simulink model "gm_flightController"  (R2018b)
settings: Solver=ode3  StartTime=0  StopTime=TFinal  FixedStep=Ts  RelTol=1e-3  EnableMultiTasking=on
libraries: hdlmdlgenlib x14
(part 2 of 2)

== system gm_flightController/Flight Controller/Yaw/Sum2 ==
  In1 : Inport
  In2 : Inport  Port=2
  Sum2 : Sum  Inputs=+-  OutDataTypeStr=single  SampleTime=0.005  SaturateOnIntegerOverflow=on  InputSameDT=on
  Out1 : Outport
  wires:
  In1/1 -> Sum2/1
  In2/1 -> Sum2/2
  Sum2/1 -> Out1/1

== system gm_flightController/Flight Controller/gravity feedforward//equilibrium thrust/D_z ==
  In1 : Inport
  In2 : Inport  Port=2
  D_z : Product  Inputs=**  OutDataTypeStr=single  SampleTime=0.005  SaturateOnIntegerOverflow=on
  Out1 : Outport
  wires:
  In1/1 -> D_z/1
  In2/1 -> D_z/2
  D_z/1 -> Out1/1

== system gm_flightController/Flight Controller/gravity feedforward//equilibrium thrust/P_z ==
  In1 : Inport
  In2 : Inport  Port=2
  P_z : Product  Inputs=**  OutDataTypeStr=single  SampleTime=0.005  SaturateOnIntegerOverflow=on
  Out1 : Outport
  wires:
  In1/1 -> P_z/1
  In2/1 -> P_z/2
  P_z/1 -> Out1/1

== system gm_flightController/Flight Controller/gravity feedforward//equilibrium thrust/SaturationThrust_LowerRelop ==
  In1 : Inport
  In2 : Inport  Port=2
  SaturationThrust_LowerRelop : RelationalOperator  Operator=>  OutDataTypeStr=boolean  SampleTime=0.005  RndMeth=Nearest
  Out1 : Outport
  wires:
  In1/1 -> SaturationThrust_LowerRelop/1
  In2/1 -> SaturationThrust_LowerRelop/2
  SaturationThrust_LowerRelop/1 -> Out1/1

== system gm_flightController/Flight Controller/gravity feedforward//equilibrium thrust/SaturationThrust_UpperRelop ==
  In1 : Inport
  In2 : Inport  Port=2
  SaturationThrust_UpperRelop : RelationalOperator  Operator=<  OutDataTypeStr=boolean  SampleTime=0.005  RndMeth=Nearest
  Out1 : Outport
  wires:
  In1/1 -> SaturationThrust_UpperRelop/1
  In2/1 -> SaturationThrust_UpperRelop/2
  SaturationThrust_UpperRelop/1 -> Out1/1

== system gm_flightController/Flight Controller/gravity feedforward//equilibrium thrust/Sum15 ==
  In1 : Inport
  In2 : Inport  Port=2
  Sum15 : Sum  Inputs=+-  OutDataTypeStr=single  SampleTime=0.005  SaturateOnIntegerOverflow=on  InputSameDT=on
  Out1 : Outport
  wires:
  In1/1 -> Sum15/1
  In2/1 -> Sum15/2
  Sum15/1 -> Out1/1

== system gm_flightController/Flight Controller/gravity feedforward//equilibrium thrust/Sum3 ==
  In1 : Inport
  In2 : Inport  Port=2
  Sum3 : Sum  Inputs=+-  OutDataTypeStr=single  SampleTime=0.005  SaturateOnIntegerOverflow=on  InputSameDT=on
  Out1 : Outport
  wires:
  In1/1 -> Sum3/1
  In2/1 -> Sum3/2
  Sum3/1 -> Out1/1

== system gm_flightController/Flight Controller/gravity feedforward//equilibrium thrust/Sum4 ==
  In1 : Inport
  In2 : Inport  Port=2
  Sum4 : Sum  OutDataTypeStr=single  SampleTime=0.005  SaturateOnIntegerOverflow=on  InputSameDT=on
  Out1 : Outport
  wires:
  In1/1 -> Sum4/1
  In2/1 -> Sum4/2
  Sum4/1 -> Out1/1

== system gm_flightController/Flight Controller/thrustsToMotorCommands/MotorDirections ==
  In1 : Inport
  MotorDirections : Gain  Gain=single([1 -1 1 -1]).'
  Out1 : Outport
  wires:
  In1/1 -> MotorDirections/1
  MotorDirections/1 -> Out1/1

== system gm_flightController/Flight Controller/thrustsToMotorCommands/Saturation5_LowerRelop ==
  In1 : Inport
  In2 : Inport  Port=2
  Saturation5_LowerRelop : RelationalOperator  Operator=>  OutDataTypeStr=boolean  SampleTime=0.005  RndMeth=Nearest
  Out1 : Outport
  wires:
  In1/1 -> Saturation5_LowerRelop/1
  In2/1 -> Saturation5_LowerRelop/2
  Saturation5_LowerRelop/1 -> Out1/1

== system gm_flightController/Flight Controller/thrustsToMotorCommands/Saturation5_UpperRelop ==
  In1 : Inport
  In2 : Inport  Port=2
  Saturation5_UpperRelop : RelationalOperator  Operator=<  OutDataTypeStr=boolean  SampleTime=0.005  RndMeth=Nearest
  Out1 : Outport
  wires:
  In1/1 -> Saturation5_UpperRelop/1
  In2/1 -> Saturation5_UpperRelop/2
  Saturation5_UpperRelop/1 -> Out1/1

== system gm_flightController/Flight Controller/thrustsToMotorCommands/ThrustToMotorCommand ==
  In1 : Inport
  In2 : Inport  Port=2
  ThrustToMotorCommand : Product  Inputs=**  OutDataTypeStr=single  SampleTime=0.005
  Out1 : Outport
  wires:
  In1/1 -> ThrustToMotorCommand/1
  In2/1 -> ThrustToMotorCommand/2
  ThrustToMotorCommand/1 -> Out1/1
